simulink model "for_using_forSubsystem"  (R2021a)
settings: Solver=VariableStepAuto  StartTime=0.0  StopTime=10.0  RelTol=1e-3
settings Model: Creator=Acer  LastModifiedBy=Acer

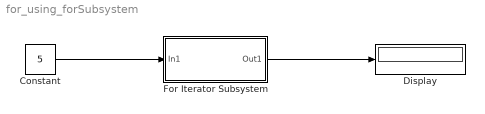
== system for_using_forSubsystem ==
  Constant : Constant  Value=5
  Display : Display
  For Iterator Subsystem : Subsystem  TreatAsAtomicUnit=on
  wires:
  Constant/1 -> For Iterator Subsystem/1(In1)
  For Iterator Subsystem/1(Out1) -> Display/1

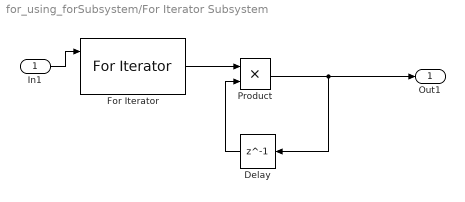
== system for_using_forSubsystem/For Iterator Subsystem ==
  In1 : Inport
  Delay : Delay  DelayLength=1  InitialCondition=1
  For Iterator : ForIterator  IterationSource=external  ExternalIncrement=on
  Product : Product  OutDataTypeStr=int32
  Out1 : Outport
  wires:
  In1/1 -> For Iterator/1
  For Iterator/1 -> Product/1
  Product/1 -> Delay/1, Out1/1
  Delay/1 -> Product/2
